simulink model "PID_conditional_AW_B"  (R2015b)
settings: Solver=VariableStepAuto  StartTime=0.0  StopTime=10.0  RelTol=1e-3
undefined symbols (not defined in the file): D_B, I_B, N_B, P_B, sat_lim_max_B, sat_lim_min_B
settings Model: Creator=mgreiff  LastModifiedBy=mgreiff

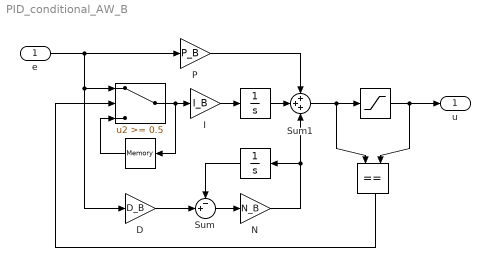
== system PID_conditional_AW_B ==
  e : Inport
  " " : Integrator
  "  " : Saturate  UpperLimit=sat_lim_max_B  LowerLimit=sat_lim_min_B
  "   " : Integrator
  "    " : Memory
  "     " : Switch  Threshold=0.5
  "       " : RelationalOperator  Operator===  OutDataTypeStr=boolean
  D : Gain  Gain=D_B
  I : Gain  Gain=I_B
  N : Gain  Gain=N_B
  P : Gain  Gain=P_B
  Sum : Sum  Inputs=-+|
  Sum1 : Sum  Inputs=+++
  u : Outport
  wires:
  e/1 -> D/1, "     "/1, P/1
  D/1 -> Sum/2
  Sum/1 -> N/1
  I/1 -> " "/1
  N/1 -> "   "/1, Sum1/3
  "   "/1 -> Sum/1
  P/1 -> Sum1/1
  " "/1 -> Sum1/2
  "    "/1 -> "     "/3
  "       "/1 -> "     "/2
  "     "/1 -> "    "/1, I/1
  Sum1/1 -> "  "/1, "       "/1
  "  "/1 -> "       "/2, u/1
